simulink model "mcb_host_encoder"  (R2022b)
settings: Solver=FixedStepDiscrete  StartTime=0.0  StopTime=inf  RelTol=1e-3  EnableMultiTasking=on
values from neighbouring files (symbols this model uses):
  PU_System = mcb_SetPUSystem(pmsm,inverter)    [mcb_pmsm_foc_qep_dsPIC33_data.m]
  Ts = T_pwm    (= 5e-05)    [mcb_pmsm_foc_qep_dsPIC33_data.m]
libraries: instrumentseriallib x2, simulink x1
settings Model: Creator=The MathWorks, Inc.  LastModifiedBy=I52209
settings SolverCC: AlgebraicLoopSolver=TrustRegion
settings DataIOCC: LimitDataPoints=on  SaveFormat=Array  ReturnWorkspaceOutputs=off
settings OptimizationCC: LifeSpan=1  EfficientTunableParamExpr=on
settings DebuggingCC: MergeDetectMultiDrivingBlocksExec=none  SolverPrmCheckMsg=warning  ParameterPrecisionLossMsg=none  UnconnectedInputMsg=warning  UnconnectedOutputMsg=warning  UnconnectedLineMsg=warning  AllowSymbolicDim=off  PregeneratedLibrarySubsystemCodeDiagnostic=none  SFUnexpectedBacktrackingDiag=warning  SFNoUnconditionalDefaultTransitionDiag=warning  SFExecutionAtInitializationDiag=none  SFMachineParentedDataDiag=warning  ArithmeticOperatorsInVariantConditions=warning
settings HardwareCC: ProdBitPerPointer=32  ProdLargestAtomicFloat=None  ProdIntDivRoundTo=Undefined  ProdEndianess=Unspecified  ProdWordSize=32  ProdHWDeviceType=32-bit Generic
settings ModelReferenceCC: EnableRefExpFcnMdlSchedulingChecks=on  PropagateSignalLabelsOutOfModel=off
settings SFSimCC: SimUseLocalCustomCode=off  MATLABDynamicMemAlloc=off
settings RTWCC: Description=Real-Time Workshop Embedded Coder  SystemTargetFile=ert.tlc  TemplateMakefile=ert_default_tmf  GenerateReport=on  RTWUseLocalCustomCode=off  IncludeHyperlinkInReport=on  LaunchReport=on  GenerateTraceInfo=on  GenerateTraceReport=on  GenerateTraceReportSl=on  GenerateTraceReportSf=on  GenerateTraceReportEml=on  DLArmComputeVersion=19.05
settings CodeAppCC: IgnoreCustomStorageClasses=off  StateflowObjectComments=on  InternalIdentifier=Classic
settings ERTTargetCC: MultiwordLength=2048  GenerateSampleERTMain=on  ERTCustomFileTemplate=example_file_process.tlc  ConvertIfToSwitch=off  SuppressUnreachableDefaultCases=off
settings ConfigComp: CovMetricSettings=dw  CovSaveCumulativeToWorkspaceVar=on  CovSaveSingleToWorkspaceVar=on  CovExternalEMLEnable=off  CovSFcnEnable=off

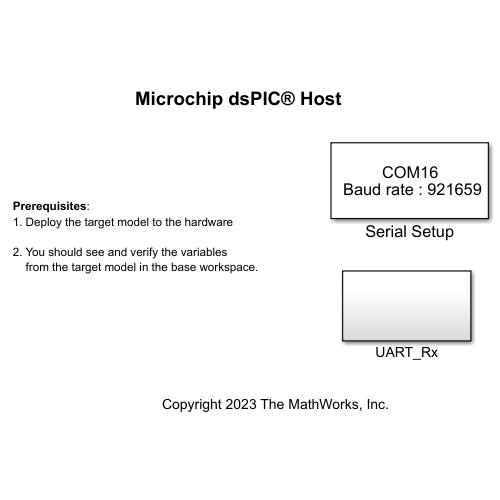
[thumbnail: Simulink's stored preview of the top-level diagram]
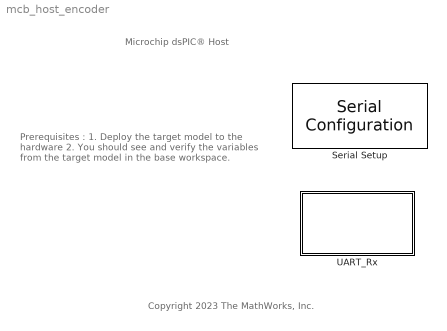
== system mcb_host_encoder ==
  note: Prerequisites :
      | 1. Deploy the target model to the hardware
      |
      | 2. You should see and verify the variables
      | from the target model in the base workspace.
  note: Microchip dsPIC® Host
  note: Copyright 2023 The MathWorks, Inc.
  Serial Setup : instrumentseriallib/Serial Configuration  Priority=-99  PortSel=COM16  Port=COM16  ComPort=COM16  BaudRate=921659  DataBits=8  Parity=none  StopBits=1  ByteOrder=little-endian  FlowControl=none  Timeout=2  SimulateUsing=Interpreted execution  BlockInModel=on  aMode=5
  UART_Rx : Subsystem

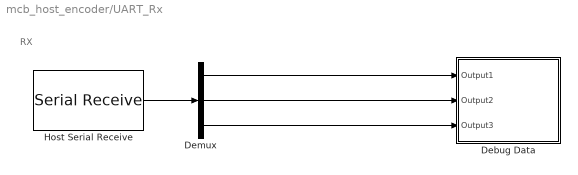
== system mcb_host_encoder/UART_Rx ==
  note: RX
  Debug Data : Subsystem
  Demux : Demux  Outputs=3
  Host Serial Receive : instrumentseriallib/Serial Receive  PortSel=COM16  Port=COM16  ComPort=COM16  DataType=uint8  SaveDataType=uint8  ToggleHeader=on  Header='S'  ToggleTerminator=on  Terminator=Custom terminator  CustomTerminator='E'  InputFormat=Row major  ToggleDataSize=on  DataSize=3  EnableBlockingMode=on  ActionDataUnavailable=Output custom value  ActionWhenDataUnavailable=Output custom value  CustomValue=15  SampleTime=Ts*100  SimulateUsing=Interpreted execution  BlockInModel=on  aMode=5
  wires:
  Demux/2 -> Debug Data/2(Output2)
  Demux/1 -> Debug Data/1(Output1)
  Host Serial Receive/1 -> Demux/1
  Demux/3 -> Debug Data/3(Output3)

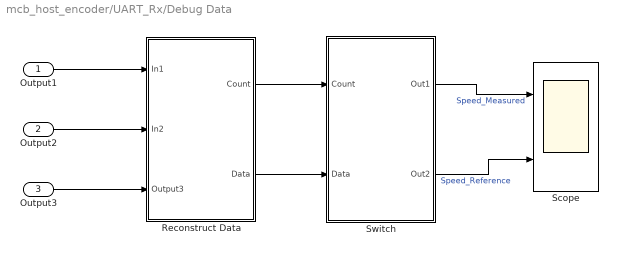
== system mcb_host_encoder/UART_Rx/Debug Data ==
  Output1 : Inport
  Output2 : Inport  Port=2
  Output3 : Inport  Port=3
  Reconstruct Data : Subsystem
  Scope : Scope  NumInputPorts=2
  Switch : Subsystem
  wires:
  Switch/2(Out2) -> Scope/2  "Speed_Reference"
  Switch/1(Out1) -> Scope/1  "Speed_Measured"
  Reconstruct Data/1(Count) -> Switch/1(Count)
  Output2/1 -> Reconstruct Data/2(In2)
  Output1/1 -> Reconstruct Data/1(In1)
  Output3/1 -> Reconstruct Data/3(Output3)
  Reconstruct Data/2(Data) -> Switch/2(Data)

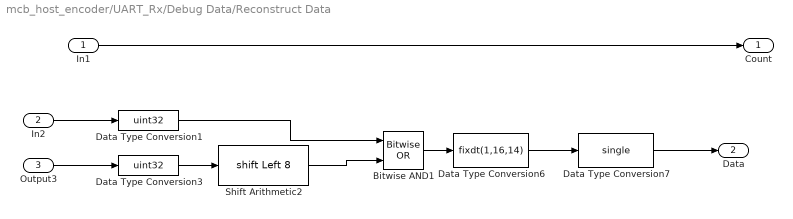
== system mcb_host_encoder/UART_Rx/Debug Data/Reconstruct Data ==
  In1 : Inport
  In2 : Inport  Port=2
  Output3 : Inport  Port=3
  Bitwise AND1 : simulink/Logic and Bit Operations/Bitwise Operator  logicop=OR  UseBitMask=off  NumInputPorts=2  BitMask=bin2dec('11011001')  BitMaskRealWorld=Stored Integer
  Data Type Conversion1 : DataTypeConversion  OutDataTypeStr=uint32  RndMeth=Simplest  SaturateOnIntegerOverflow=off
  Data Type Conversion3 : DataTypeConversion  OutDataTypeStr=uint32  RndMeth=Simplest  SaturateOnIntegerOverflow=off
  Data Type Conversion6 : DataTypeConversion  OutDataTypeStr=fixdt(1,16,14)  ConvertRealWorld=Stored Integer (SI)  RndMeth=Simplest  SaturateOnIntegerOverflow=off
  Data Type Conversion7 : DataTypeConversion  OutDataTypeStr=single  RndMeth=Simplest  SaturateOnIntegerOverflow=off
  Shift Arithmetic2 : ArithShift  BitShiftNumber=8  BitShiftDirection=Left
  Count : Outport
  Data : Outport  Port=2
  wires:
  In1/1 -> Count/1
  Data Type Conversion1/1 -> Bitwise AND1/1
  Bitwise AND1/1 -> Data Type Conversion6/1
  Shift Arithmetic2/1 -> Bitwise AND1/2
  Data Type Conversion7/1 -> Data/1
  Data Type Conversion6/1 -> Data Type Conversion7/1
  In2/1 -> Data Type Conversion1/1
  Data Type Conversion3/1 -> Shift Arithmetic2/1
  Output3/1 -> Data Type Conversion3/1

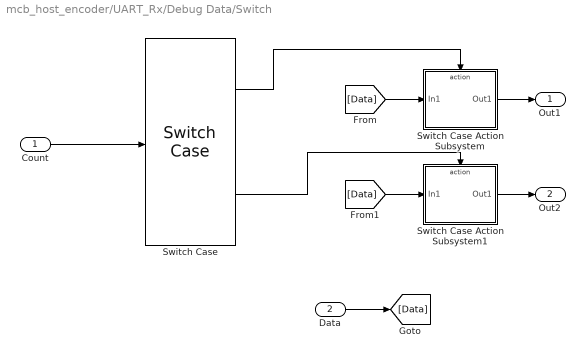
== system mcb_host_encoder/UART_Rx/Debug Data/Switch ==
  Count : Inport
  Data : Inport  Port=2
  Switch Case : SwitchCase  CaseConditions={0,1}  ShowDefaultCase=off
  Switch Case Action Subsystem : Subsystem  TreatAsAtomicUnit=on
  Switch Case Action Subsystem1 : Subsystem  TreatAsAtomicUnit=on
  Out1 : Outport
  Out2 : Outport  Port=2
  wires:
  [Data] -> Switch Case Action Subsystem/1(In1)
  Switch Case Action Subsystem/1(Out1) -> Out1/1
  Switch Case/2 -> Switch Case Action Subsystem1/Action
  [Data] -> Switch Case Action Subsystem1/1(In1)
  Data/1 -> [Data]
  Count/1 -> Switch Case/1
  Switch Case Action Subsystem1/1(Out1) -> Out2/1
  Switch Case/1 -> Switch Case Action Subsystem/Action

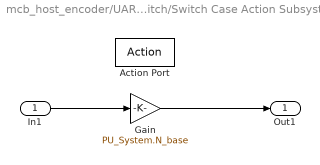
== system mcb_host_encoder/UART_Rx/Debug Data/Switch/Switch Case Action Subsystem ==
  In1 : Inport
  Action Port : ActionPort  ActionPortLabel=case [ 0 ]:
  Gain : Gain  Gain=PU_System.N_base
  Out1 : Outport
  wires:
  Gain/1 -> Out1/1
  In1/1 -> Gain/1

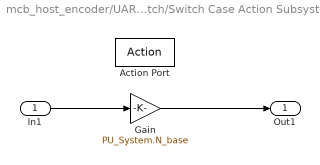
== system mcb_host_encoder/UART_Rx/Debug Data/Switch/Switch Case Action Subsystem1 ==
  In1 : Inport
  Action Port : ActionPort  ActionPortLabel=case [ 1 ]:
  Gain : Gain  Gain=PU_System.N_base
  Out1 : Outport
  wires:
  Gain/1 -> Out1/1
  In1/1 -> Gain/1
